simulink model "IS_O"  (Simulink 7.9)
settings: Solver=ode45  StartTime=0.0  StopTime=50  FixedStep=0.001  RelTol=1e-3
settings Model: Creator=compiaffe  LastModifiedBy=compiaffe

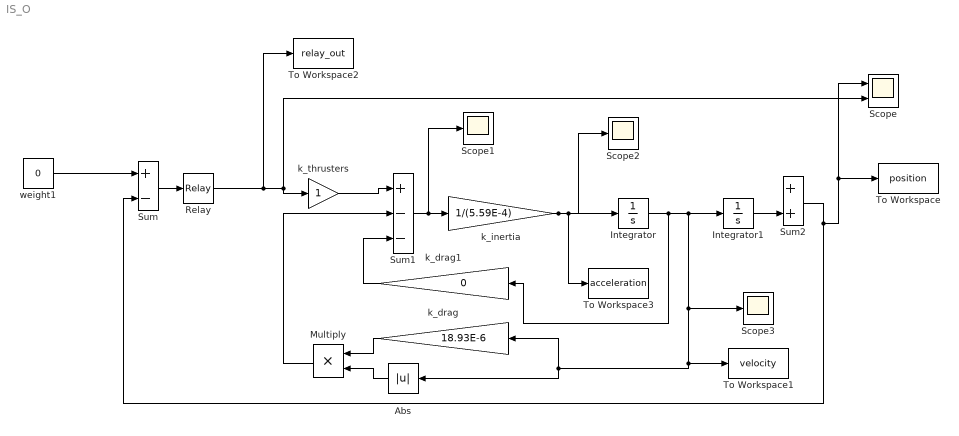
== system IS_O ==
  Abs : Abs
  Integrator : Integrator
  Integrator1 : Integrator
  Multiply : Product  Inputs=**
  Relay : Relay  OnSwitchValue=22.5  OffSwitchValue=-22.5  OnOutputValue=17.09E-2  OffOutputValue=-17.09E-2
  Scope : Scope  NumInputPorts=2
      settings: TickLabels=on  ShowLegends=on  YMin=-2e-12~-2.3205  YMax=-1e-13~-2.0995  SampleTime=1
  Scope1 : Scope
      settings: TimeRange=0.16
  Scope2 : Scope
      settings: TimeRange=0.16  SaveName=ScopeData2
  Scope3 : Scope
      settings: TimeRange=0.16  SaveName=ScopeData3
  Sum : Sum  Inputs=+-
  Sum1 : Sum  Inputs=+--
  Sum2 : Sum
  To Workspace : ToWorkspace  VariableName=position  SampleTime=-1  SaveFormat=Timeseries
  To Workspace1 : ToWorkspace  VariableName=velocity  SampleTime=-1  SaveFormat=Timeseries
  To Workspace2 : ToWorkspace  VariableName=relay_out  SampleTime=-1  SaveFormat=Timeseries
  To Workspace3 : ToWorkspace  VariableName=acceleration  SampleTime=-1  SaveFormat=Timeseries
  k_drag : Gain  Gain=18.93E-6
  k_drag1 : Gain  Gain=0
  k_inertia : Gain  Gain=1/(5.59E-4)
  k_thrusters : Gain
  weight1 : Constant  Value=0
  wires:
  Sum/1 -> Relay/1
  Integrator/1 -> Integrator1/1, Scope3/1, k_drag/1, Abs/1, To Workspace1/1, k_drag1/1
  weight1/1 -> Sum/1
  Integrator1/1 -> Sum2/2
  Sum2/1 -> Sum/2, Scope/1, To Workspace/1
  Relay/1 -> k_thrusters/1, Scope/2, To Workspace2/1
  k_drag/1 -> Multiply/1
  Multiply/1 -> Sum1/2
  k_thrusters/1 -> Sum1/1
  Sum1/1 -> k_inertia/1, Scope1/1
  k_inertia/1 -> Integrator/1, Scope2/1, To Workspace3/1
  Abs/1 -> Multiply/2
  k_drag1/1 -> Sum1/3
